simulink model "svm_oloop"  (Simulink 8.6)
settings: Solver=FixedStepAuto  StartTime=0.0  StopTime=10.0  FixedStep=uavsim.svm.tsample_model  RelTol=1e-3
libraries: svm_lib x1
settings Model: Creator=j.bolting  LastModifiedBy=j.bolting
settings DataIOCC: SaveFormat=Dataset  SignalLoggingSaveFormat=Dataset
settings OptimizationCC: ExpressionDepthLimit=128
settings DebuggingCC: UnderspecifiedInitializationDetection=Simplified  MergeDetectMultiDrivingBlocksExec=error  SolverPrmCheckMsg=none  FcnCallInpInsideContextMsg=EnableAllAsError  StateNameClashWarn=none
settings HardwareCC: ProdBitPerPointer=64  ProdLargestAtomicFloat=Float  ProdIntDivRoundTo=Zero  ProdEndianess=LittleEndian  ProdWordSize=64  ProdHWDeviceType=Intel->x86-64 (Windows64)
settings GRTTargetCC: GeneratePreprocessorConditionals=Use local settings  CombineOutputUpdateFcns=on  GRTInterface=off
settings ConfigComp: CovModelRefEnable=off

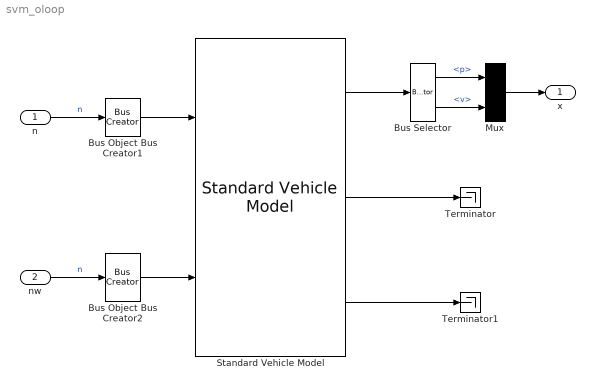
== system svm_oloop ==
  n : Inport  PortDimensions=3
  nw : Inport  Port=2  PortDimensions=3
  Bus Selector : BusSelector  OutputSignals=p,v
  Bus Object Bus Creator1 : BusCreator  Inputs=1  OutDataTypeStr=Bus: svm_bus_u  mask(BUS OBJECT Bus Creator){busType=Bus: svm_bus_u}
      mask prompts: busType "Bus Type"
      mask help:
      | Provides users the cabability to painlessly, instantly customize bus creators of output data type 'Bus:' by selecting the bus object type from a drop down menu dynamically populated by bus objects in the workspace.
      |
      | After pressing the "Apply Selection" button signal lines into the creator are populated and named with the elements in the chosen bus saving the user from having to recall and fill out signal line names.
      |
      | NOTE that when copying a Bus Object Bus Creator from your locked Library the link to the Library is automatically broken. This saves the user from having to Unlock Links To Library (From the Library menu.), Disable Link and finally Break Link (Both from the Model menu.) for every placed instance of the block.
      settings: AttributesFormatString=%<OutDataTypeStr>  CopyFcn=set_param(gcb, 'LinkStatus', 'none')
      mask TypeOptions busType: Bus: Acceleration | Bus: Aero | Bus: Airframe | Bus: Attitude | Bus: CMD | Bus: Environment | Bus: FlightGearData | Bus: Kinematics | Bus: Position | Bus: RotationalAcceleration | Bus: RotationalVelocity | Bus: Velocity | Bus: svm_bus_d_exo | Bus: svm_bus_u | Bus: svm_bus_x | Bus: svm_bus_xi
      mask Callback busType:
      | % Using variable names terminated with "_BOBC" to lessen the chances of
      | % collisions with existing workspace variables.
      | 
      | % Get the current block handle and mask handle.
      | handleCreator_BOBC = gcbh;
      | maskObj_BOBC       = Simulink.Mask.get(gcb);
      | 
      | % Get a list of variables in the workspace in order to search for the '1x1
      | % Bus' types.
      | wsVars_BOBC = whos;
      | 
      | % Reset the 'TypeOptions' bus list in case some '1x1 Bus' types have been
      | % deleted from or added to the workspace.
      | maskObj_BOBC.Parameters.TypeOptions = {'<empty>'};
      | 
      | % Reset the bus count.
      | busCount_BOBC = 0;
      | 
      | for index_BOBC = 1:length(wsVars_BOBC)
      | 
      |    % If the variable is a bus object...
      |    if strcmp(wsVars_BOBC(index_BOBC).class, 'Simulink.Bus')
      | 
      |       busCount_BOBC = busCount_BOBC + 1;
      | 
      |       % ... add it to the TypeOptions of the mask.
      |       maskObj_BOBC.Parameters.TypeOptions(busCount_BOBC) = ...
      |                                                            ...
      |                                  {['Bus: ', wsVars_BOBC(index_BOBC).name]};
      |    end
      | end
      | 
      | if busCount_BOBC == 0
      | 
      |    % If there are NO bus objects in the workspace then provide a warning
      |    % popup...
      |    warndlg('There are currently no bus objects in the workspace - you have no use for this block. Use a normal Bus Creator instead.')
      | 
      |    % ... and do nothing.
      | elseif ~strcmp(get_param(handleCreator_BOBC, 'OutDataTypeStr'), 'Inherit: auto')
      | 
      |    % If the currently selected bus data type ('OutDataTypeStr') is not
      |    % 'Inherit: auto' (i.e., if we are reopening the mask.) then get the
      |    % current 'OutDataTypeStr' and 'maskVal.' ('maskVal' is the selected
      |    % 'TypeOptions' list member.)
      |    outDatStr_BOBC = get_param(handleCreator_BOBC, 'OutDataTypeStr');
      |    maskVal_BOBC   = get_param(handleCreator_BOBC, 'MaskValues');
      | 
      |    if ~strcmp(outDatStr_BOBC, maskVal_BOBC{1})
      | 
      |       % Upon re-opening the mask if the default 'TypeOptions' list member
      |       % (The first one.) contained in 'maskVal' does not match the
      |       % currently selected bus data type ('OutDataTypeStr') then set the
      |       % 'TypeOptions' list member to the selected bus data type. (Cuts down
      |       % on confusion to have the displayed list member match the selected
      |       % bus data type rather than the first entry.)
      |       set_param(handleCreator_BOBC, 'MaskValues', {outDatStr_BOBC});
      |    end
      | end
      | 
      | % Clean up the workspace.
      | clear  handleCreator_BOBC  maskObj_BOBC     wsVars_BOBC ...
      |             busCount_BOBC    index_BOBC  outDatStr_BOBC ...
      |              maskVal_BOBC
      mask DialogControl applyMOCBSelection Prompt: Apply Selection
      mask DialogControl applyMOCBSelection Callback:
      | % Using variable names terminated with "_BOBC" to lessen the chances of
      | % collisions with existing workspace variables.
      | 
      | % Get the current block, current block handle and mask handle.
      | currentBlock_BOBC  = gcb;
      | handleCreator_BOBC = gcbh;
      | 
      | % Get the desired bus type...
      | desiredBusType_BOBC = get_param(handleCreator_BOBC, 'busType');
      | 
      | % ... and set the 'OutDataTypeStr' to it.
      | set_param(handleCreator_BOBC, 'OutDataTypeStr', desiredBusType_BOBC);
      | 
      | %% First delete any existing lines on the port.
      | % Get the line handles.
      | lh_BOBC = get_param(handleCreator_BOBC, 'LineHandles');
      | 
      | % If any lines exist (Non- -1 line handles.), delete them and start over.
      | if max(lh_BOBC.Inport > 0)
      | 
      |    for index_BOBC = 1:length(lh_BOBC.Inport)
      | 
      |       if lh_BOBC.Inport(index_BOBC) > 0
      | 
      |          delete_line(lh_BOBC.Inport(index_BOBC))
      |       end
      |    end
      | end
      | 
      | %% Then work on adding new lines.
      | 
      | % Get the block path for 'add_line' function.
      | blockPath_BOBC = get_param(handleCreator_BOBC, 'Parent');
      | 
      | % Get the newly selected bus type ('OutDataTypeStr')...
      | mocbBusType_BOBC = get_param(currentBlock_BOBC, 'OutDataTypeStr');
      | 
      | % ... and parse off "Bus: " so the string of the desired bus contained in
      | % 'OutDataTypeStr' matches the raw workspace bus names.
      | mocbBusType_BOBC = mocbBusType_BOBC(6:end);
      | 
      | % Then evaluate the string containing the workspace bus name which will
      | % load the desired bus parameters.
      | busParams_BOBC = eval(mocbBusType_BOBC);
      | 
      | % From the parameters grab the number of lines to add.
      | numLines_BOBC = length(busParams_BOBC.Elements);
      | 
      | % Set the number of inputs of the masked bus creator to the number of lines
      | % to add.
      | set_param(handleCreator_BOBC, 'Inputs', num2str(numLines_BOBC));
      | 
      | % Get (Inputs.) port handles so we can grab the positions of them.
      | ph_BOBC = get_param(handleCreator_BOBC, 'PortHandles');
      | 
      | for index_BOBC = 1:numLines_BOBC
      | 
      |    % Get the position of input port number 'index_BOBC'.
      |    portPos_BOBC = get_param(ph_BOBC.Inport(index_BOBC), 'Position');
      | 
      |    % Add a line from 50 pixels left of the port position to the port
      |    % position. (This must be done because it's the lines that get named,
      |    % not the port positions.)
      |    portLine_BOBC = add_line(blockPath_BOBC, [portPos_BOBC - [50 0]; portPos_BOBC]);
      | 
      |    % Rename the new line to the bus 'index_BOBC-st/nd/rd/th' element name.
      |    set_param(portLine_BOBC, 'Name', busParams_BOBC.Elements(index_BOBC).Name)
      | end
      | 
      | %% Cleanup the workspace.
      | clear    currentBlock_BOBC  handleCreator_BOBC      index_BOBC ...
      |        desiredBusType_BOBC             lh_BOBC  blockPath_BOBC ...
      |           mocbBusType_BOBC      busParams_BOBC   numLines_BOBC ...
      |                    ph_BOBC        portPos_BOBC   portLine_BOBC
  Bus Object Bus Creator2 : BusCreator  Inputs=1  OutDataTypeStr=Bus: svm_bus_u  mask(BUS OBJECT Bus Creator){busType=Bus: svm_bus_u}
      mask prompts: busType "Bus Type"
      mask help:
      | Provides users the cabability to painlessly, instantly customize bus creators of output data type 'Bus:' by selecting the bus object type from a drop down menu dynamically populated by bus objects in the workspace.
      |
      | After pressing the "Apply Selection" button signal lines into the creator are populated and named with the elements in the chosen bus saving the user from having to recall and fill out signal line names.
      |
      | NOTE that when copying a Bus Object Bus Creator from your locked Library the link to the Library is automatically broken. This saves the user from having to Unlock Links To Library (From the Library menu.), Disable Link and finally Break Link (Both from the Model menu.) for every placed instance of the block.
      settings: AttributesFormatString=%<OutDataTypeStr>  CopyFcn=set_param(gcb, 'LinkStatus', 'none')
      mask TypeOptions busType: Bus: Acceleration | Bus: Aero | Bus: Airframe | Bus: Attitude | Bus: CMD | Bus: Environment | Bus: FlightGearData | Bus: Kinematics | Bus: Position | Bus: RotationalAcceleration | Bus: RotationalVelocity | Bus: Velocity | Bus: svm_bus_d_exo | Bus: svm_bus_u | Bus: svm_bus_x | Bus: svm_bus_xi
      mask Callback busType:
      | % Using variable names terminated with "_BOBC" to lessen the chances of
      | % collisions with existing workspace variables.
      | 
      | % Get the current block handle and mask handle.
      | handleCreator_BOBC = gcbh;
      | maskObj_BOBC       = Simulink.Mask.get(gcb);
      | 
      | % Get a list of variables in the workspace in order to search for the '1x1
      | % Bus' types.
      | wsVars_BOBC = whos;
      | 
      | % Reset the 'TypeOptions' bus list in case some '1x1 Bus' types have been
      | % deleted from or added to the workspace.
      | maskObj_BOBC.Parameters.TypeOptions = {'<empty>'};
      | 
      | % Reset the bus count.
      | busCount_BOBC = 0;
      | 
      | for index_BOBC = 1:length(wsVars_BOBC)
      | 
      |    % If the variable is a bus object...
      |    if strcmp(wsVars_BOBC(index_BOBC).class, 'Simulink.Bus')
      | 
      |       busCount_BOBC = busCount_BOBC + 1;
      | 
      |       % ... add it to the TypeOptions of the mask.
      |       maskObj_BOBC.Parameters.TypeOptions(busCount_BOBC) = ...
      |                                                            ...
      |                                  {['Bus: ', wsVars_BOBC(index_BOBC).name]};
      |    end
      | end
      | 
      | if busCount_BOBC == 0
      | 
      |    % If there are NO bus objects in the workspace then provide a warning
      |    % popup...
      |    warndlg('There are currently no bus objects in the workspace - you have no use for this block. Use a normal Bus Creator instead.')
      | 
      |    % ... and do nothing.
      | elseif ~strcmp(get_param(handleCreator_BOBC, 'OutDataTypeStr'), 'Inherit: auto')
      | 
      |    % If the currently selected bus data type ('OutDataTypeStr') is not
      |    % 'Inherit: auto' (i.e., if we are reopening the mask.) then get the
      |    % current 'OutDataTypeStr' and 'maskVal.' ('maskVal' is the selected
      |    % 'TypeOptions' list member.)
      |    outDatStr_BOBC = get_param(handleCreator_BOBC, 'OutDataTypeStr');
      |    maskVal_BOBC   = get_param(handleCreator_BOBC, 'MaskValues');
      | 
      |    if ~strcmp(outDatStr_BOBC, maskVal_BOBC{1})
      | 
      |       % Upon re-opening the mask if the default 'TypeOptions' list member
      |       % (The first one.) contained in 'maskVal' does not match the
      |       % currently selected bus data type ('OutDataTypeStr') then set the
      |       % 'TypeOptions' list member to the selected bus data type. (Cuts down
      |       % on confusion to have the displayed list member match the selected
      |       % bus data type rather than the first entry.)
      |       set_param(handleCreator_BOBC, 'MaskValues', {outDatStr_BOBC});
      |    end
      | end
      | 
      | % Clean up the workspace.
      | clear  handleCreator_BOBC  maskObj_BOBC     wsVars_BOBC ...
      |             busCount_BOBC    index_BOBC  outDatStr_BOBC ...
      |              maskVal_BOBC
      mask DialogControl applyMOCBSelection Prompt: Apply Selection
      mask DialogControl applyMOCBSelection Callback:
      | % Using variable names terminated with "_BOBC" to lessen the chances of
      | % collisions with existing workspace variables.
      | 
      | % Get the current block, current block handle and mask handle.
      | currentBlock_BOBC  = gcb;
      | handleCreator_BOBC = gcbh;
      | 
      | % Get the desired bus type...
      | desiredBusType_BOBC = get_param(handleCreator_BOBC, 'busType');
      | 
      | % ... and set the 'OutDataTypeStr' to it.
      | set_param(handleCreator_BOBC, 'OutDataTypeStr', desiredBusType_BOBC);
      | 
      | %% First delete any existing lines on the port.
      | % Get the line handles.
      | lh_BOBC = get_param(handleCreator_BOBC, 'LineHandles');
      | 
      | % If any lines exist (Non- -1 line handles.), delete them and start over.
      | if max(lh_BOBC.Inport > 0)
      | 
      |    for index_BOBC = 1:length(lh_BOBC.Inport)
      | 
      |       if lh_BOBC.Inport(index_BOBC) > 0
      | 
      |          delete_line(lh_BOBC.Inport(index_BOBC))
      |       end
      |    end
      | end
      | 
      | %% Then work on adding new lines.
      | 
      | % Get the block path for 'add_line' function.
      | blockPath_BOBC = get_param(handleCreator_BOBC, 'Parent');
      | 
      | % Get the newly selected bus type ('OutDataTypeStr')...
      | mocbBusType_BOBC = get_param(currentBlock_BOBC, 'OutDataTypeStr');
      | 
      | % ... and parse off "Bus: " so the string of the desired bus contained in
      | % 'OutDataTypeStr' matches the raw workspace bus names.
      | mocbBusType_BOBC = mocbBusType_BOBC(6:end);
      | 
      | % Then evaluate the string containing the workspace bus name which will
      | % load the desired bus parameters.
      | busParams_BOBC = eval(mocbBusType_BOBC);
      | 
      | % From the parameters grab the number of lines to add.
      | numLines_BOBC = length(busParams_BOBC.Elements);
      | 
      | % Set the number of inputs of the masked bus creator to the number of lines
      | % to add.
      | set_param(handleCreator_BOBC, 'Inputs', num2str(numLines_BOBC));
      | 
      | % Get (Inputs.) port handles so we can grab the positions of them.
      | ph_BOBC = get_param(handleCreator_BOBC, 'PortHandles');
      | 
      | for index_BOBC = 1:numLines_BOBC
      | 
      |    % Get the position of input port number 'index_BOBC'.
      |    portPos_BOBC = get_param(ph_BOBC.Inport(index_BOBC), 'Position');
      | 
      |    % Add a line from 50 pixels left of the port position to the port
      |    % position. (This must be done because it's the lines that get named,
      |    % not the port positions.)
      |    portLine_BOBC = add_line(blockPath_BOBC, [portPos_BOBC - [50 0]; portPos_BOBC]);
      | 
      |    % Rename the new line to the bus 'index_BOBC-st/nd/rd/th' element name.
      |    set_param(portLine_BOBC, 'Name', busParams_BOBC.Elements(index_BOBC).Name)
      | end
      | 
      | %% Cleanup the workspace.
      | clear    currentBlock_BOBC  handleCreator_BOBC      index_BOBC ...
      |        desiredBusType_BOBC             lh_BOBC  blockPath_BOBC ...
      |           mocbBusType_BOBC      busParams_BOBC   numLines_BOBC ...
      |                    ph_BOBC        portPos_BOBC   portLine_BOBC
  Mux : Mux  Inputs=2
  Standard Vehicle Model : svm_lib/Standard Vehicle Model  mask_p0_NED=[0 0 0]  mask_v0_NED=[15 0 0]
  Terminator : Terminator
  Terminator1 : Terminator
  x : Outport
  wires:
  Standard Vehicle Model/1 -> Bus Selector/1
  Bus Object Bus Creator1/1 -> Standard Vehicle Model/1
  Bus Selector/2 -> Mux/2  "<v>"
  Bus Selector/1 -> Mux/1  "<p>"
  Mux/1 -> x/1
  Bus Object Bus Creator2/1 -> Standard Vehicle Model/2
  Standard Vehicle Model/2 -> Terminator/1
  Standard Vehicle Model/3 -> Terminator1/1
  nw/1 -> Bus Object Bus Creator2/1  "n"
  n/1 -> Bus Object Bus Creator1/1  "n"
